simulink model "planta_con_pid"  (R2025a)
settings: Solver=VariableStepAuto  StartTime=0.0  StopTime=100  RelTol=1e-3
values from neighbouring files (symbols this model uses):
  B = 1.812642814729166e-04    (= 0.000181264281473)    [PI_calculo.m]    (also in anterior.m = 0.00181520669083; datos_planta.m = 0.00181520669083; definir_incertidumbre.m = ureal('B', 1.81e-4, 'Percentage', 20); hallar_PID.m = 0.00181520669083)
  I = 0.0362    [PI_calculo.m]    (also in anterior.m = 0.0361594958333; datos_planta.m = 0.0361594958333; definir_incertidumbre.m = ureal('I', 0.0362 , 'Percentage', 15); hallar_PID.m = 0.0361594958333)
  k = (m*g*l/(2*I) + m_adicional * g * l / I)    (= 0.872324904512)    [anterior.m]    (also in datos_planta.m; hallar_PID.m; planta_procedimiento.m)
  K_pwm_F = 0.0002    [anterior.m]    (also in datos_planta.m; planta_procedimiento.m)
  K_rad_grados = 180 / pi    (= 57.2957795131)    [anterior.m]    (also in datos_planta.m; planta_procedimiento.m)
  Kp = 10    [PI_calculo.m]    (also in datos_planta.m; definir_incertidumbre.m; hallar_PID.m = 1; planta_procedimiento.m)
  l = 0.145    [anterior.m]    (also in datos_planta.m; hallar_PID.m; planta_procedimiento.m)
libraries: slpidlib x1
settings Model: Creator=sergi  LastModifiedBy=sergi

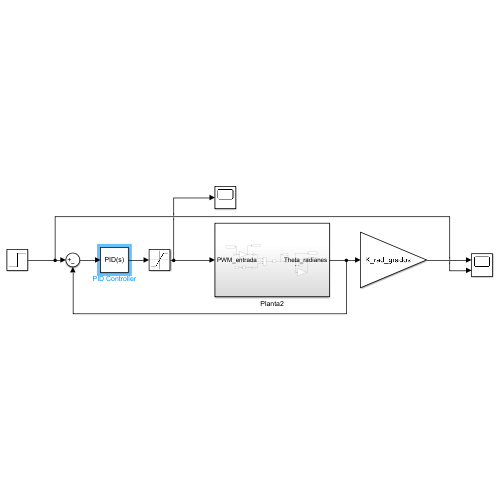
[thumbnail: Simulink's stored preview of the top-level diagram]
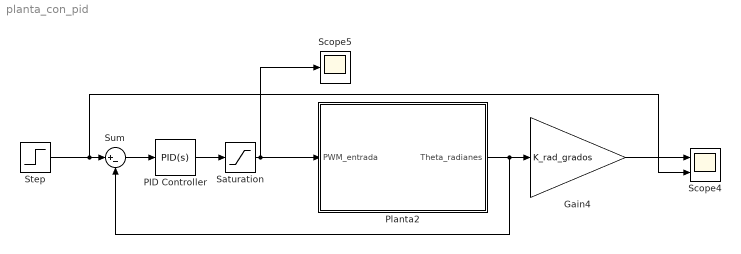
== system planta_con_pid ==
  Gain4 : Gain  Gain=K_rad_grados
  PID Controller : slpidlib/PID Controller  Controller=PID  Form=Parallel  TimeDomain=Continuous-time  UseExternalTs=off  SampleTime=-1  IntegratorMethod=Forward Euler  FilterMethod=Forward Euler  ControllerParametersSource=internal  P=Kp  I=0  UseKiTs=off  D=0  UseExternalDerivativeSource=off  N=100  UseFilter=on  TunerSelectOption=Transfer Function Based (PID Tuner App)  InitialConditionSource=internal  InitialConditionForIntegrator=0  InitialConditionForFilter=0  DifferentiatorICPrevScaledInput=0  ExternalReset=none  TrackingMode=off  Kt=1  LimitOutput=off  SatLimitsSource=internal  UpperSaturationLimit=inf  LowerSaturationLimit=-inf  LinearizeAsGain=on  AntiWindupMode=none  Kb=1  LimitIntegrator=off  UpperIntegratorSaturationLimit=inf  LowerIntegratorSaturationLimit=-inf  POutMin=[]  POutMax=[]  IOutMin=[]  IOutMax=[]  DOutMin=[]  DOutMax=[]  NOutMin=[]  NOutMax=[]  SumOutMin=[]  SumOutMax=[]  SaturationOutMin=[]  SaturationOutMax=[]  PParamMin=[]  PParamMax=[]  IParamMin=[]  IParamMax=[]  DParamMin=[]  DParamMax=[]  NParamMin=[]  NParamMax=[]  KbParamMin=[]  KbParamMax=[]  KtParamMin=[]  KtParamMax=[]  KbOutMin=[]  KbOutMax=[]  KtOutMin=[]  KtOutMax=[]  IntegratorOutMin=[]  IntegratorOutMax=[]  FilterOutMin=[]  FilterOutMax=[]  SumI1OutMin=[]  SumI1OutMax=[]  SumI2OutMin=[]  SumI2OutMax=[]  SumI3OutMin=[]  SumI3OutMax=[]  SumI4OutMin=[]  SumI4OutMax=[]  SumDOutMin=[]  SumDOutMax=[]  DifferentiatorOutMin=[]  DifferentiatorOutMax=[]  FilterDiffOutCoefMin=[]  FilterDiffOutCoefMax=[]  ReciprocalOutMin=[]  ReciprocalOutMax=[]  SumDenOutMin=[]  SumDenOutMax=[]  SumNumOutMin=[]  SumNumOutMax=[]  DivideOutMin=[]  DivideOutMax=[]  UdiffTsProdOutMin=[]  UdiffTsProdOutMax=[]  NTsProdOutMin=[]  NTsProdOutMax=[]  UintegralTsProdOutMin=[]  UintegralTsProdOutMax=[]  UngainTsProdOutMin=[]  UngainTsProdOutMax=[]  ClampingZeroOutDataTypeStr=Inherit: Inherit via back propagation  ClampingZeroOutMin=[]  ClampingZeroOutMax=[]  FilterDenConstantOutDataTypeStr=Inherit: Inherit via back propagation  FilterDenConstantOutMin=[]  FilterDenConstantOutMax=[]  PCopyOutDataTypeStr=Inherit: Inherit via back propagation  PCopyOutMin=[]  PCopyOutMax=[]  NCopyOutDataTypeStr=Inherit: Inherit via back propagation  NCopyOutMin=[]  NCopyOutMax=[]  IntegratorContinuousStateAttributes=''  IntegratorStateMustResolveToSignalObject=off  IntegratorRTWStateStorageClass=Auto  FilterContinuousStateAttributes=''  FilterStateMustResolveToSignalObject=off  FilterRTWStateStorageClass=Auto  ParallelPVariant=InternalParameters  IdealPVariant=Disabled  IVariant=InternalParameters  DVariant=InternalParameters  IntegratorVariant=Continuous  SatVariant=Disabled  AWVariant=Passthrough  PCopyVariant=Disabled  TRVariant=Disabled  FdbkBlocksVariant=Forward  IdealPFdbkVariant=Disabled  SatFdbkVariant=Disabled  DerivativeFilterVariant=ContFilter  NVariant=InternalParameters  NCopyVariant=Disabled  FilterICVariant=InternalICsFilter  IntegratorICVariant=InternalICs  ExternalResetVariant=Disabled  TRSumVariant=Passthrough  SumFdbkVariant=Disabled  SumVariant=Sum_PID  TsampFilterVariant=InternalTs  TsampNgainVariant=Passthrough  TsampIntegralVariant=Disabled_SignalSpec  ExternalSaturationOutDataTypeStr=Inherit: Same as second input  DerivativeSourceVariant=ErrorSignal  PreIntVariant=InternalPreInt
  Planta2 : Subsystem
  Saturation : Saturate  UpperLimit=1025  LowerLimit=0
  Scope4 : Scope  NumInputPorts=2
      settings: ActiveDisplayYMinimum=-20.61734395011354  ActiveDisplayYMaximum=68.118997704139417  DataLoggingVariableName=ScopeData4
  Scope5 : Scope
      settings: ActiveDisplayYMinimum=-165.09356618749939  ActiveDisplayYMaximum=1278.8055452241183  DataLoggingVariableName=ScopeData5
  Step : Step  Time=10  After=30  SampleTime=0
  Sum : Sum  Inputs=|+-
  wires:
  Sum/1 -> PID Controller/1
  Step/1 -> Scope4/2, Sum/1
  PID Controller/1 -> Saturation/1
  Planta2/1(Theta_radianes) -> Sum/2, Gain4/1
  Saturation/1 -> Planta2/1(PWM_entrada), Scope5/1
  Gain4/1 -> Scope4/1

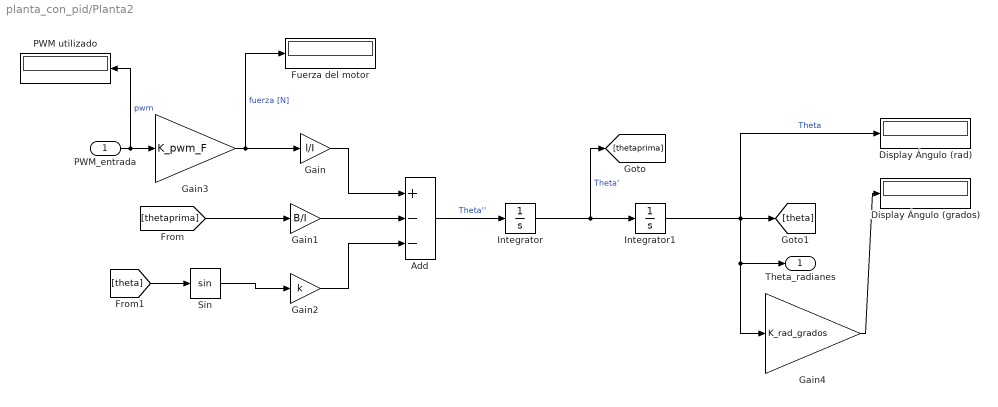
== system planta_con_pid/Planta2 ==
  PWM_entrada : Inport
  Add : Sum  Inputs=+--
  Display Ángulo (grados) : Display
  Display Ángulo (rad) : Display
  Fuerza del motor : Display
  Gain : Gain  Gain=l/I
  Gain1 : Gain  Gain=B/I
  Gain2 : Gain  Gain=k
  Gain3 : Gain  Gain=K_pwm_F
  Gain4 : Gain  Gain=K_rad_grados
  Integrator : Integrator
  Integrator1 : Integrator
  PWM utilizado : Display
  Sin : Trigonometry
  Theta_radianes : Outport
  wires:
  Gain2/1 -> Add/3
  [thetaprima] -> Gain1/1
  Add/1 -> Integrator/1  "Theta''"
  PWM_entrada/1 -> PWM utilizado/1, Gain3/1  "pwm"
  Integrator/1 -> [thetaprima], Integrator1/1  "Theta'"
  Integrator1/1 -> Theta_radianes/1, Gain4/1, Display Ángulo (rad)/1, [theta]  "Theta"
  Gain3/1 -> Fuerza del motor/1, Gain/1  "fuerza [N]"
  Gain/1 -> Add/1
  Gain1/1 -> Add/2
  [theta] -> Sin/1
  Sin/1 -> Gain2/1
  Gain4/1 -> Display Ángulo (grados)/1
